simulink model "singele_phase_to_3phase_svpwm_IM_VF_PI"  (Simulink 10.0)
settings: Solver=ode23t  StartTime=0.0  StopTime=5  FixedStep=0.00001  MaxStep=10e-6  RelTol=1e-3  EnableMultiTasking=on
libraries: powerlib x12, powerlib_extras x2, simulink x2
settings Model: Creator=jagan  LastModifiedBy=bhisma
settings SolverCC: ZeroCrossControl=DisableAll  ZeroCrossAlgorithm=Non-adaptive
settings DataIOCC: LimitDataPoints=on  SignalLoggingSaveFormat=ModelDataLogs
settings OptimizationCC: ExpressionDepthLimit=2147483647  InitFltsAndDblsToZero=on
settings DebuggingCC: SaveWithParameterizedLinksMsg=none  SignalResolutionControl=TryResolveAllWithWarning  SolverPrmCheckMsg=warning  MultiTaskDSMMsg=warning  MultiTaskCondExecSysMsg=none  FcnCallInpInsideContextMsg=warning  StateNameClashWarn=warning
settings SFSimCC: SimUseLocalCustomCode=on  SimParseCustomCode=off  CustomCodeUndefinedFunction=FilterOut
settings RTWCC: RTWUseLocalCustomCode=on
settings GRTTargetCC: TargetFcnLib=ansi_tfl_tmw.mat

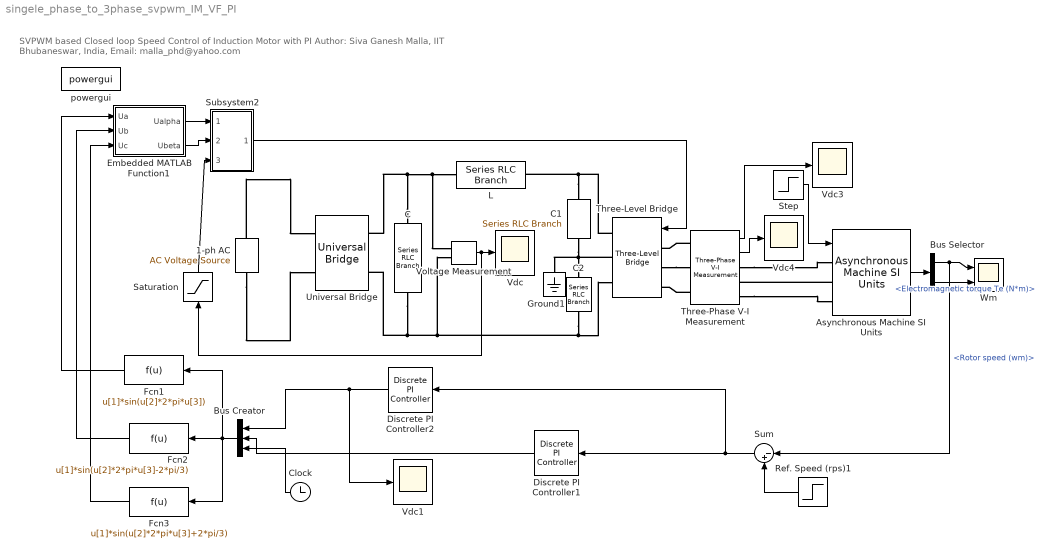
== system singele_phase_to_3phase_svpwm_IM_VF_PI ==
  note: SVPWM based  Closed loop Speed Control  of Induction Motor with PI
      | Author: Siva Ganesh Malla, IIT Bhubaneswar, India, Email: malla_phd@yahoo.com
  1-ph AC : powerlib/Electrical Sources/AC Voltage Source  SystemSampleTime=-1  Amplitude=650  Phase=0  Frequency=50  SampleTime=0  Measurements=None
      settings: SourceProductName=Simscape Electrical
  Asynchronous Machine SI Units : powerlib/Machines/Asynchronous Machine SI Units  SystemSampleTime=-1  PresetModel=No  MechanicalLoad=Torque Tm  ShowDetailedParameters=on  RotorType=Squirrel-cage  ReferenceFrame=Rotor  NominalParameters=[3730 350 50]  Stator=[1.115 0.005974]  Rotor=[1.083 0.005974]  Lm=0.2037  Mechanical=[0.02 0.005752 2]  PolePairs=2  InitialConditions="[ 1,0   0,0,0   0,0,0 ]"  Units=SI  LoadFlowParameters=0  SimulateSaturation=off  Saturation=[9.9249,19.6672,38.0377,51.3988,69.2824,105.1337,152.5532,214.2421,303.1917;230, 322, 414, 460, 506, 552, 598, 644, 690]  TsPowergui=0  TsBlock=-1
      settings: SourceProductName=Simscape Electrical
  Bus Creator : BusCreator  Inputs=3
  Bus Selector : BusSelector  OutputSignals=Mechanical.Rotor speed (wm),Mechanical.Electromagnetic torque Te (N*m)
  C : powerlib/Elements/Series RLC Branch  PhysicalDomain=powersysdomain  SubClassName=unknown  LeftPortType=p1  RightPortType=p1  LConnTagsString=__new0  RConnTagsString=__new0  BranchType=C  Resistance=1  Inductance=1e-3  SetiL0=off  InitialCurrent=0  Capacitance=10e-6  Setx0=off  InitialVoltage=0  Measurements=None
      settings: SourceProductName=Simscape Electrical
  C1 : powerlib/Elements/Series RLC Branch  PhysicalDomain=powersysdomain  SubClassName=unknown  LeftPortType=p1  RightPortType=p1  LConnTagsString=__new0  RConnTagsString=__new0  BranchType=C  Resistance=1  Inductance=1e-3  SetiL0=off  InitialCurrent=0  Capacitance=2300e-6  Setx0=off  InitialVoltage=0  Measurements=None
      settings: SourceProductName=Simscape Electrical
  C2 : powerlib/Elements/Series RLC Branch  PhysicalDomain=powersysdomain  SubClassName=unknown  LeftPortType=p1  RightPortType=p1  LConnTagsString=__new0  RConnTagsString=__new0  BranchType=C  Resistance=1  Inductance=1e-3  SetiL0=off  InitialCurrent=0  Capacitance=2300e-6  Setx0=off  InitialVoltage=0  Measurements=None
      settings: SourceProductName=Simscape Electrical
  Clock : Clock
  Discrete PI Controller1 : powerlib_extras/Discrete  Control Blocks/Discrete PI Controller  SystemSampleTime=-1  Kp=0.6  Ki=80  Par_Limits=[70 0]  Init=0  Ts=50e-6
      settings: SourceProductName=Simscape Electrical
  Discrete PI Controller2 : powerlib_extras/Discrete  Control Blocks/Discrete PI Controller  SystemSampleTime=-1  Kp=2  Ki=120  Par_Limits=[350 0]  Init=0  Ts=50e-6
      settings: SourceProductName=Simscape Electrical
  Embedded MATLAB Function1 : MATLAB Function  TreatAsAtomicUnit=on
  Fcn1 : Fcn  Expr=u[1]*sin(u[2]*2*pi*u[3])
  Fcn2 : Fcn  Expr=u[1]*sin(u[2]*2*pi*u[3]-2*pi/3)
  Fcn3 : Fcn  Expr=u[1]*sin(u[2]*2*pi*u[3]+2*pi/3)
  Ground1 : powerlib/Elements/Ground  PhysicalDomain=powersysdomain  SubClassName=unknown  LeftPortType=p1  RightPortType=p1  LConnTagsString=a
      settings: SourceProductName=Simscape Electrical
  L : powerlib/Elements/Series RLC Branch  PhysicalDomain=powersysdomain  SubClassName=unknown  LeftPortType=p1  RightPortType=p1  LConnTagsString=__new0  RConnTagsString=__new0  BranchType=L  Resistance=1  Inductance=0.1e-3  SetiL0=off  InitialCurrent=0  Capacitance=1e-6  Setx0=off  InitialVoltage=0  Measurements=None
      settings: SourceProductName=Simscape Electrical
  Ref. Speed (rps)1 : Step  Time=3  Before=157  After=130  SampleTime=0
  Saturation : Saturate  UpperLimit=750  LowerLimit=10
  Step : Step  After=3  SampleTime=0
  Subsystem2 : Subsystem
  Sum : Sum  Inputs=|-+
  Three-Level Bridge : powerlib/Power Electronics/Three-Level Bridge  SystemSampleTime=-1  Arms=3  SnubberResistance=50  SbubberCapacitance=1e-6  Device=IGBT / Diodes  Ron=0.2e-3  ForwardVoltages="[  2 1 ]"  Measurements=All voltages and currents
      settings: SourceProductName=Simscape Electrical  SourceProductBaseCode=PS
  Three-Phase V-I Measurement : powerlib/Measurements/Three-Phase V-I Measurement  SystemSampleTime=-1  VoltageMeasurement=phase-to-phase  SetLabelV=off  LabelV=Vabc  Vpu=off  CurrentMeasurement=yes  SetLabelI=off  LabelI=Iabc  Ipu=off  Pbase=100e6  Vbase=500e3  OutputType=Complex  PhasorSimulation=off  PSBequivalent=0
      settings: SourceProductName=Simscape Electrical
  Universal Bridge : powerlib/Power Electronics/Universal Bridge  SystemSampleTime=-1  Arms=2  SnubberResistance=1e5  SnubberCapacitance=inf  Device=Diodes  Ron=1e-3  Lon=0  ForwardVoltages="[  0  0  ]"  ForwardVoltage=0  GTOparameters=[ 10e-6 , 20e-6 ]  IGBTparameters=[ 1e-6 , 2e-6 ]  Measurements=None  converterType=Rectifier
      settings: SourceProductName=Simscape Electrical
  Vdc{,1,3..4} (4 alike) : Scope
  Voltage Measurement : powerlib/Measurements/Voltage Measurement  SystemSampleTime=-1  PhasorSimulation=off  OutputType=Complex  PSBequivalent=0
      settings: SourceProductName=Simscape Electrical
  Wm : Scope  NumInputPorts=2
  powergui : powerlib/powergui  SystemSampleTime=-1  SimulationMode=Discrete  SampleTime=50e-6  frequency=60  SPID=off  SwTol=0  Interpol=off  x0status=blocks  echomessages=off  HookPort=off  FunctionMessages=off  EnableUseOfTLC=off  RestoreLinks=warning  frequencyindice=50  Frange=[0:2:500]  Ylog=off  Xlog=on  ShowGrid=off  save=off  variable=ZData  ZoomFFT=on  StartTime=0.0  cycles=1  DisplayStyle=1  fundamental=60  FreqAxis=off  MaxFrequency=1000  frequencyindicesteady=1  RmsSteady=1  display=off  Ts=0  methode=off
      settings: SourceProductName=Simscape Electrical
  wires:
  Step/1 -> Asynchronous Machine SI Units/1
  Embedded MATLAB Function1/1(Ualpha) -> Subsystem2/1(Ualfa)
  Embedded MATLAB Function1/2(Ubeta) -> Subsystem2/2(Ubeta)
  Asynchronous Machine SI Units/1 -> Bus Selector/1
  Bus Selector/1 -> Wm/1, Sum/1  "<Rotor speed (wm)>"
  Bus Selector/2 -> Wm/2  "<Electromagnetic torque Te (N*m)>"
  Subsystem2/1(pulse) -> Three-Level Bridge/1
  Three-Phase V-I Measurement/1 -> Vdc3/1
  Three-Phase V-I Measurement/2 -> Vdc4/1
  Bus Creator/1 -> Fcn2/1, Fcn1/1, Fcn3/1
  Clock/1 -> Bus Creator/3
  Discrete PI Controller1/1 -> Bus Creator/2
  Fcn1/1 -> Embedded MATLAB Function1/1(Ua)
  Fcn2/1 -> Embedded MATLAB Function1/2(Ub)
  Fcn3/1 -> Embedded MATLAB Function1/3(Uc)
  Voltage Measurement/1 -> Vdc/1, Saturation/1
  Saturation/1 -> Subsystem2/3(Vdc)
  Ref. Speed (rps)1/1 -> Sum/2
  Sum/1 -> Discrete PI Controller1/1, Discrete PI Controller2/1
  Discrete PI Controller2/1 -> Bus Creator/1, Vdc1/1
  connections:
  Three-Phase V-I Measurement/LConn1 -- Three-Level Bridge/LConn1
  Three-Level Bridge/LConn2 -- Three-Phase V-I Measurement/LConn2
  Three-Phase V-I Measurement/LConn3 -- Three-Level Bridge/LConn3
  Three-Phase V-I Measurement/RConn1 -- Asynchronous Machine SI Units/LConn1
  Asynchronous Machine SI Units/LConn2 -- Three-Phase V-I Measurement/RConn2
  Three-Phase V-I Measurement/RConn3 -- Asynchronous Machine SI Units/LConn3
  C/LConn1 -- L/LConn1 -- Voltage Measurement/LConn1 -- Universal Bridge/RConn1
  Three-Level Bridge/RConn3 -- C2/RConn1 -- Voltage Measurement/LConn2 -- Universal Bridge/RConn2 -- C/RConn1
  C1/LConn1 -- Three-Level Bridge/RConn1 -- L/RConn1
  Ground1/LConn1 -- C1/RConn1 -- C2/LConn1 -- Three-Level Bridge/RConn2
  1-ph AC/RConn1 -- Universal Bridge/LConn1
  1-ph AC/LConn1 -- Universal Bridge/LConn2

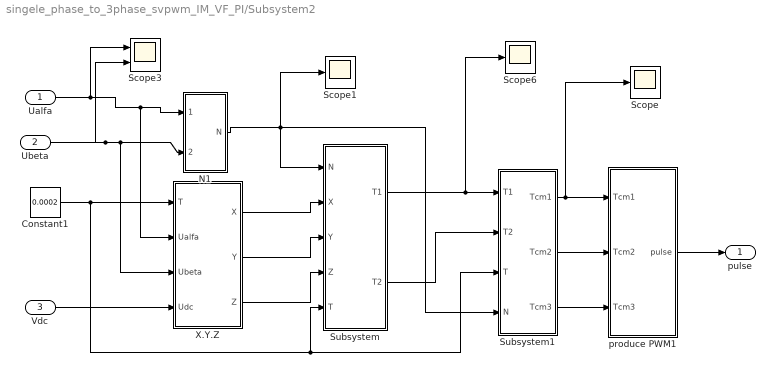
== system singele_phase_to_3phase_svpwm_IM_VF_PI/Subsystem2 ==
  Ualfa : Inport
  Ubeta : Inport  Port=2
  Vdc : Inport  Port=3
  Constant1 : Constant  Value=0.0002
  N1 : Subsystem
  Scope : Scope
  Scope1 : Scope
  Scope3 : Scope  NumInputPorts=2
  Scope6 : Scope
  Subsystem : Subsystem
  Subsystem1 : Subsystem
  X.Y.Z : Subsystem
  produce PWM1 : Subsystem
  pulse : Outport
  wires:
  Constant1/1 -> X.Y.Z/1(T), Subsystem1/3(T), Subsystem/5(T)
  Vdc/1 -> X.Y.Z/4(Udc)
  N1/1(N) -> Subsystem1/4(N), Scope1/1, Subsystem/1(N)
  X.Y.Z/1(X) -> Subsystem/2(X)
  X.Y.Z/2(Y) -> Subsystem/3(Y)
  X.Y.Z/3(Z) -> Subsystem/4(Z)
  Subsystem1/1(Tcm1) -> Scope/1, produce PWM1/1(Tcm1)
  Subsystem1/2(Tcm2) -> produce PWM1/2(Tcm2)
  Subsystem1/3(Tcm3) -> produce PWM1/3(Tcm3)
  Ualfa/1 -> Scope3/1, X.Y.Z/2(Ualfa), N1/1(Ualfa)
  Subsystem/1(T1) -> Subsystem1/1(T1), Scope6/1
  Subsystem/2(T2) -> Subsystem1/2(T2)
  Ubeta/1 -> N1/2(Ubeta), X.Y.Z/3(Ubeta), Scope3/2
  produce PWM1/1(pulse) -> pulse/1

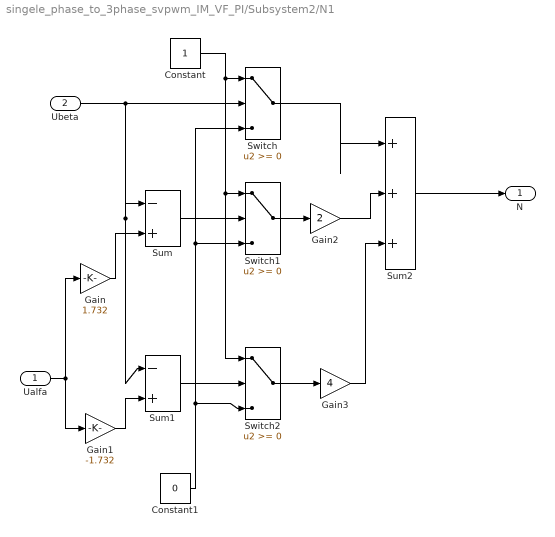
== system singele_phase_to_3phase_svpwm_IM_VF_PI/Subsystem2/N1 ==
  Ualfa : Inport
  Ubeta : Inport  Port=2
  Constant : Constant
  Constant1 : Constant  Value=0
  Gain : Gain  Gain=1.732
  Gain1 : Gain  Gain=-1.732
  Gain2 : Gain  Gain=2
  Gain3 : Gain  Gain=4
  Sum : Sum  Inputs=|-+
  Sum1 : Sum  Inputs=|-+
  Sum2 : Sum  Inputs=|+++
  Switch : Switch
  Switch1 : Switch
  Switch2 : Switch
  N : Outport
  wires:
  Ubeta/1 -> Switch/2, Sum/1, Sum1/1
  Constant/1 -> Switch/1, Switch2/1, Switch1/1
  Ualfa/1 -> Gain1/1, Gain/1
  Gain/1 -> Sum/2
  Sum/1 -> Switch1/2
  Sum1/1 -> Switch2/2
  Gain1/1 -> Sum1/2
  Constant1/1 -> Switch/3, Switch1/3, Switch2/3
  Switch1/1 -> Gain2/1
  Switch2/1 -> Gain3/1
  Gain2/1 -> Sum2/2
  Switch/1 -> Sum2/1
  Gain3/1 -> Sum2/3
  Sum2/1 -> N/1

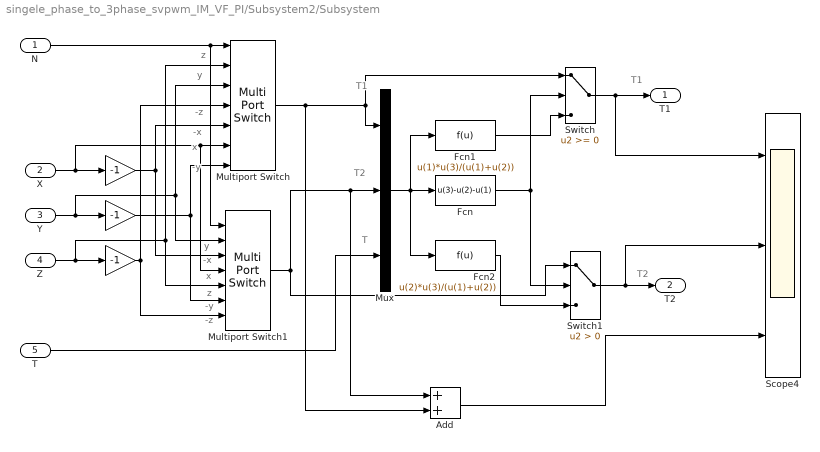
== system singele_phase_to_3phase_svpwm_IM_VF_PI/Subsystem2/Subsystem ==
  note: z
  note: y
  note: -z
  note: -x
  note: x
  note: -y
  note: y
  note: -x
  note: x
  note: z
  note: -y
  note: -z
  note: T1
  note: T2
  note: T
  note: T1
  note: T2
  N : Inport
  X : Inport  Port=2
  Y : Inport  Port=3
  Z : Inport  Port=4
  T : Inport  Port=5
  " " : Gain  Gain=-1
  "  " : Gain  Gain=-1
  "    " : Gain  Gain=-1
  Add : Sum
  Fcn : Fcn  Expr=u(3)-u(2)-u(1)
  Fcn1 : Fcn  Expr=u(1)*u(3)/(u(1)+u(2))
  Fcn2 : Fcn  Expr=u(2)*u(3)/(u(1)+u(2))
  Multiport Switch : MultiPortSwitch  Inputs=6
  Multiport Switch1 : MultiPortSwitch  Inputs=6
  Mux : Mux  Inputs=3
  Scope4 : Scope  NumInputPorts=3
  Switch : Switch
  Switch1 : Switch  Criteria=u2 > Threshold
  T1 : Outport
  T2 : Outport  Port=2
  wires:
  N/1 -> Multiport Switch1/1, Multiport Switch/1
  X/1 -> Multiport Switch1/4, Multiport Switch/6, " "/1
  Y/1 -> Multiport Switch1/2, Multiport Switch/3, "  "/1
  Z/1 -> Multiport Switch1/5, Multiport Switch/2, "    "/1
  "    "/1 -> Multiport Switch1/7, Multiport Switch/4
  "  "/1 -> Multiport Switch/7, Multiport Switch1/6
  " "/1 -> Multiport Switch/5, Multiport Switch1/3
  Multiport Switch/1 -> Mux/1, Switch/1, Add/2
  Multiport Switch1/1 -> Switch1/1, Mux/2, Add/1
  T/1 -> Mux/3
  Mux/1 -> Fcn/1, Fcn1/1, Fcn2/1
  Fcn/1 -> Switch/2, Switch1/2
  Fcn1/1 -> Switch/3
  Fcn2/1 -> Switch1/3
  Switch/1 -> T1/1, Scope4/1
  Switch1/1 -> T2/1, Scope4/2
  Add/1 -> Scope4/3

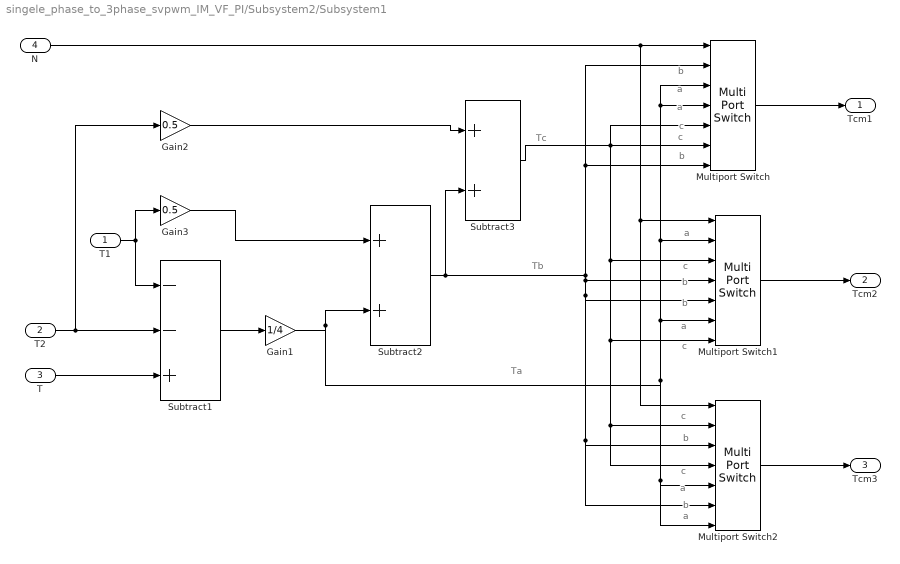
== system singele_phase_to_3phase_svpwm_IM_VF_PI/Subsystem2/Subsystem1 ==
  note: Ta
  note: Tb
  note: Tc
  note: b
  note: a
  note: a
  note: c
  note: c
  note: b
  note: a
  note: c
  note: b
  note: b
  note: a
  note: c
  note: c
  note: b
  note: c
  note: a
  note: b
  note: a
  T1 : Inport
  T2 : Inport  Port=2
  T : Inport  Port=3
  N : Inport  Port=4
  Gain1 : Gain  Gain=1/4
  Gain2 : Gain  Gain=0.5
  Gain3 : Gain  Gain=0.5
  Multiport Switch : MultiPortSwitch  Inputs=6
  Multiport Switch1 : MultiPortSwitch  Inputs=6
  Multiport Switch2 : MultiPortSwitch  Inputs=6
  Subtract1 : Sum  Inputs=--+
  Subtract2 : Sum
  Subtract3 : Sum
  Tcm1 : Outport
  Tcm2 : Outport  Port=2
  Tcm3 : Outport  Port=3
  wires:
  T2/1 -> Gain2/1, Subtract1/2
  T/1 -> Subtract1/3
  T1/1 -> Gain3/1, Subtract1/1
  Gain3/1 -> Subtract2/1
  Subtract1/1 -> Gain1/1
  Gain1/1 -> Subtract2/2, Multiport Switch/3, Multiport Switch/4, Multiport Switch1/2, Multiport Switch1/6, Multiport Switch2/5, Multiport Switch2/7
  Subtract2/1 -> Subtract3/2, Multiport Switch/2, Multiport Switch/7, Multiport Switch1/4, Multiport Switch1/5, Multiport Switch2/3, Multiport Switch2/6
  Gain2/1 -> Subtract3/1
  N/1 -> Multiport Switch/1, Multiport Switch2/1, Multiport Switch1/1
  Multiport Switch/1 -> Tcm1/1
  Multiport Switch1/1 -> Tcm2/1
  Multiport Switch2/1 -> Tcm3/1
  Subtract3/1 -> Multiport Switch/5, Multiport Switch/6, Multiport Switch1/3, Multiport Switch1/7, Multiport Switch2/2, Multiport Switch2/4

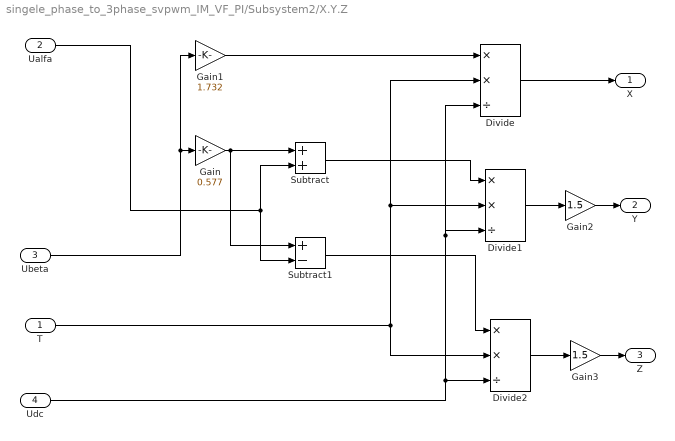
== system singele_phase_to_3phase_svpwm_IM_VF_PI/Subsystem2/X.Y.Z ==
  T : Inport
  Ualfa : Inport  Port=2
  Ubeta : Inport  Port=3
  Udc : Inport  Port=4
  Divide : Product  Inputs=**/
  Divide1 : Product  Inputs=**/
  Divide2 : Product  Inputs=**/
  Gain : Gain  Gain=0.577
  Gain1 : Gain  Gain=1.732
  Gain2 : Gain  Gain=1.5
  Gain3 : Gain  Gain=1.5
  Subtract : Sum
  Subtract1 : Sum  Inputs=+-
  X : Outport
  Y : Outport  Port=2
  Z : Outport  Port=3
  wires:
  Gain/1 -> Subtract/1, Subtract1/1
  Gain1/1 -> Divide/1
  T/1 -> Divide2/2, Divide1/2, Divide/2
  Udc/1 -> Divide2/3, Divide1/3, Divide/3
  Ualfa/1 -> Subtract1/2, Subtract/2
  Subtract/1 -> Divide1/1
  Subtract1/1 -> Divide2/1
  Divide/1 -> X/1
  Divide1/1 -> Gain2/1
  Divide2/1 -> Gain3/1
  Gain2/1 -> Y/1
  Gain3/1 -> Z/1
  Ubeta/1 -> Gain1/1, Gain/1

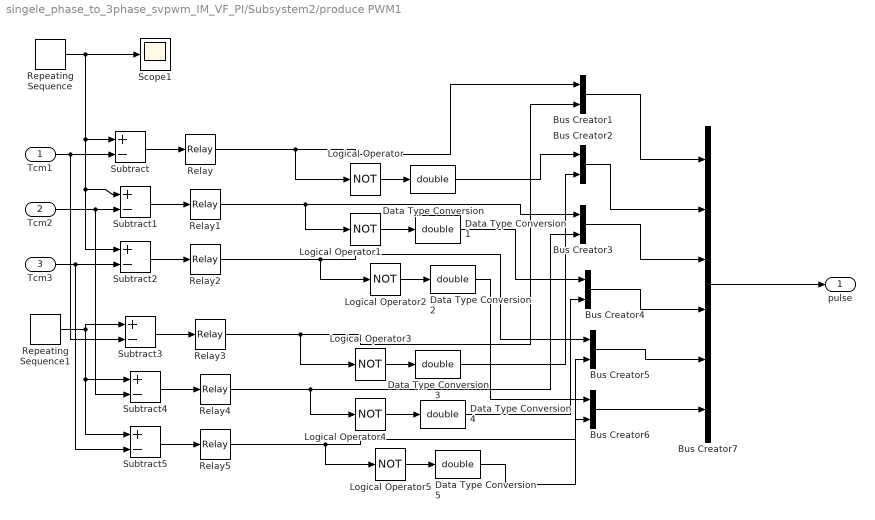
== system singele_phase_to_3phase_svpwm_IM_VF_PI/Subsystem2/produce PWM1 ==
  Tcm1 : Inport
  Tcm2 : Inport  Port=2
  Tcm3 : Inport  Port=3
  Bus Creator{1..6} (6 alike) : BusCreator  Inputs=2
  Bus Creator7 : BusCreator  Inputs=6
  Data Type Conversion{,1..5} (6 alike) : DataTypeConversion  OutDataTypeStr=double
  Logical Operator{,1..5} (6 alike) : Logic  Operator=NOT  AllPortsSameDT=off
  Relay{,1..5} (6 alike) : Relay
  Repeating Sequence : simulink/Sources/Repeating Sequence  SystemSampleTime=-1  rep_seq_t=[0 0.0001 0.0002]  rep_seq_y=[0 0.0001/2 0]
  Repeating Sequence1 : simulink/Sources/Repeating Sequence  SystemSampleTime=-1  rep_seq_t=[0 0.0001 0.0002]  rep_seq_y=[0.0001/2 0.0001 0.0001/2]
  Scope1 : Scope
  Subtract{,1..5} (6 alike) : Sum  Inputs=+-
  pulse : Outport
  wires:
  Data Type Conversion2/1 -> Bus Creator6/1
  Data Type Conversion1/1 -> Bus Creator4/1
  Data Type Conversion/1 -> Bus Creator2/1
  Relay2/1 -> Logical Operator2/1, Bus Creator5/1
  Relay1/1 -> Logical Operator1/1, Bus Creator3/1
  Relay/1 -> Logical Operator/1, Bus Creator1/1
  Logical Operator/1 -> Data Type Conversion/1
  Logical Operator2/1 -> Data Type Conversion2/1
  Logical Operator1/1 -> Data Type Conversion1/1
  Tcm3/1 -> Subtract2/2, Subtract5/2
  Tcm2/1 -> Subtract1/2, Subtract4/2
  Tcm1/1 -> Subtract/2, Subtract3/2
  Repeating Sequence/1 -> Scope1/1, Subtract1/1, Subtract2/1, Subtract/1
  Subtract2/1 -> Relay2/1
  Subtract1/1 -> Relay1/1
  Subtract/1 -> Relay/1
  Subtract5/1 -> Relay5/1
  Subtract4/1 -> Relay4/1
  Subtract3/1 -> Relay3/1
  Repeating Sequence1/1 -> Subtract3/1, Subtract4/1, Subtract5/1
  Data Type Conversion5/1 -> Bus Creator6/2
  Data Type Conversion4/1 -> Bus Creator4/2
  Data Type Conversion3/1 -> Bus Creator2/2
  Relay5/1 -> Logical Operator5/1, Bus Creator5/2
  Relay4/1 -> Logical Operator4/1, Bus Creator3/2
  Relay3/1 -> Logical Operator3/1, Bus Creator1/2
  Logical Operator3/1 -> Data Type Conversion3/1
  Logical Operator5/1 -> Data Type Conversion5/1
  Logical Operator4/1 -> Data Type Conversion4/1
  Bus Creator1/1 -> Bus Creator7/1
  Bus Creator2/1 -> Bus Creator7/2
  Bus Creator3/1 -> Bus Creator7/3
  Bus Creator4/1 -> Bus Creator7/4
  Bus Creator5/1 -> Bus Creator7/5
  Bus Creator6/1 -> Bus Creator7/6
  Bus Creator7/1 -> pulse/1

== matlab function Embedded MATLAB Function1 ==
  settings: fimath=|
      | fimath(...
      | 'RoundMode', 'floor',...
      | 'OverflowMode', 'wrap',...
      | 'ProductMode', 'KeepLSB', 'ProductWordLength', 32,...
      | 'SumMode', 'KeepLSB', 'SumWordLength', 32,...
      | 'CastBeforeSum', false)
  data: Ua input double; Ualpha output double; Ub input double; Uc input double; Ubeta output double
function [Ualpha,Ubeta]= fcn(Ua,Ub,Uc)
% This block supports an embeddable subset of the MATLAB language.
% See the help menu for details. 

Ualpha=2/3*(Ua-0.5*Ub-0.5*Uc);
Ubeta=2/3*(sqrt(3)/2*Ub-sqrt(3)/2*Uc);
